simulink model "quadplane_controlA"  (R2023a)
settings: Solver=VariableStepAuto  StartTime=0.0  StopTime=10.0  RelTol=1e-3
undefined symbols (not defined in the file or in its folder): framePeriod_s
libraries: simulink x4
settings Model: Creator=lagerprocessor  LastModifiedBy=lagerprocessor

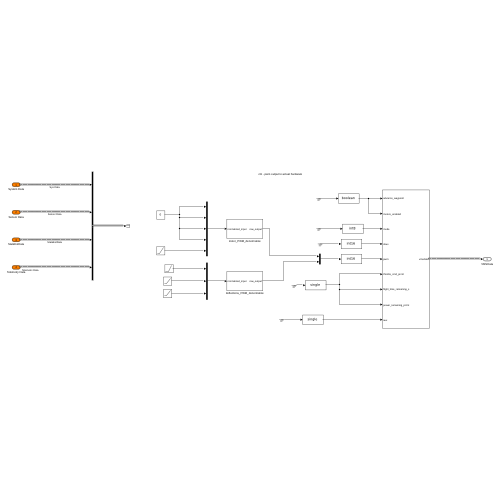
[thumbnail: Simulink's stored preview of the top-level diagram]
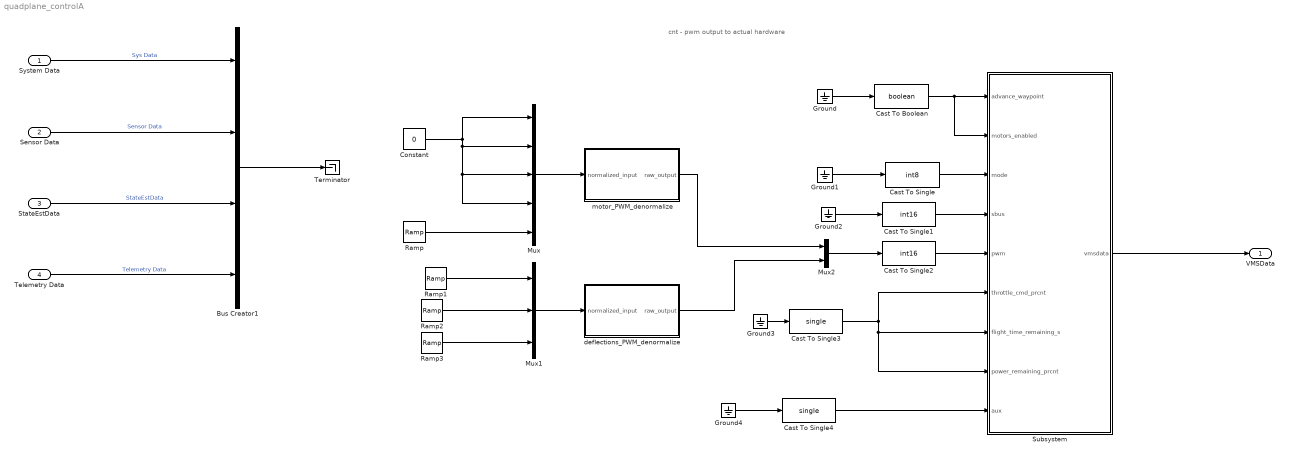
== system quadplane_controlA ==
  note: cnt - pwm output to actual hardware
  System Data : Inport  OutDataTypeStr=Bus: SysData  SampleTime=framePeriod_s  BusOutputAsStruct=on
  Sensor Data : Inport  Port=2  OutDataTypeStr=Bus: SensorData  SampleTime=framePeriod_s  BusOutputAsStruct=on
  StateEstData : Inport  Port=3  OutDataTypeStr=Bus: StateEstData  SampleTime=framePeriod_s  BusOutputAsStruct=on
  Telemetry Data : Inport  Port=4  OutDataTypeStr=Bus: TelemData  SampleTime=framePeriod_s  BusOutputAsStruct=on
  Bus Creator1 : BusCreator  Inputs=4
  Cast To Boolean : DataTypeConversion  OutDataTypeStr=boolean  SaturateOnIntegerOverflow=off  RndMeth=Floor
  Cast To Single : DataTypeConversion  OutDataTypeStr=int8  SaturateOnIntegerOverflow=off  RndMeth=Floor
  Cast To Single1 : DataTypeConversion  OutDataTypeStr=int16  SaturateOnIntegerOverflow=off  RndMeth=Floor
  Cast To Single2 : DataTypeConversion  OutDataTypeStr=int16  SaturateOnIntegerOverflow=off  RndMeth=Floor
  Cast To Single3 : DataTypeConversion  OutDataTypeStr=single  SaturateOnIntegerOverflow=off  RndMeth=Floor
  Cast To Single4 : DataTypeConversion  OutDataTypeStr=single  SaturateOnIntegerOverflow=off  RndMeth=Floor
  Constant : Constant  Value=0
  Ground{,1..4} (5 alike) : Ground
  Mux : Mux  Inputs=5
  Mux1 : Mux  Inputs=3
  Mux2 : Mux  Inputs=2
  Ramp : simulink/Sources/Ramp  slope=0  start=0  InitialOutput=0.4
  Ramp1 : simulink/Sources/Ramp  slope=0  start=0  InitialOutput=0
  Ramp2 : simulink/Sources/Ramp  slope=0  start=0  InitialOutput=0
  Ramp3 : simulink/Sources/Ramp  slope=0  start=0  InitialOutput=0
  Subsystem : Subsystem
  Terminator : Terminator
  deflections_PWM_denormalize : Subsystem
  motor_PWM_denormalize : Subsystem
  VMSData : Outport  OutDataTypeStr=Bus: VmsData
  wires:
  Telemetry Data/1 -> Bus Creator1/4  "Telemetry Data"
  StateEstData/1 -> Bus Creator1/3  "StateEstData"
  Sensor Data/1 -> Bus Creator1/2  "Sensor Data"
  System Data/1 -> Bus Creator1/1  "Sys Data"
  Bus Creator1/1 -> Terminator/1
  motor_PWM_denormalize/1(raw_output) -> Mux2/1
  Ground/1 -> Cast To Boolean/1
  Ground1/1 -> Cast To Single/1
  Ground2/1 -> Cast To Single1/1
  Cast To Single3/1 -> Subsystem/6(throttle_cmd_prcnt), Subsystem/8(power_remaining_prcnt), Subsystem/7(flight_time_remaining_s)
  Cast To Single4/1 -> Subsystem/9(aux)
  Subsystem/1(vmsdata) -> VMSData/1
  Cast To Boolean/1 -> Subsystem/2(motors_enabled), Subsystem/1(advance_waypoint)
  Cast To Single/1 -> Subsystem/3(mode)
  Cast To Single1/1 -> Subsystem/4(sbus)
  Cast To Single2/1 -> Subsystem/5(pwm)
  Ground3/1 -> Cast To Single3/1
  Ground4/1 -> Cast To Single4/1
  Mux/1 -> motor_PWM_denormalize/1(normalized_input)
  Ramp/1 -> Mux/5
  Constant/1 -> Mux/4, Mux/3, Mux/2, Mux/1
  Mux1/1 -> deflections_PWM_denormalize/1(normalized_input)
  deflections_PWM_denormalize/1(raw_output) -> Mux2/2
  Mux2/1 -> Cast To Single2/1
  Ramp3/1 -> Mux1/3
  Ramp2/1 -> Mux1/2
  Ramp1/1 -> Mux1/1

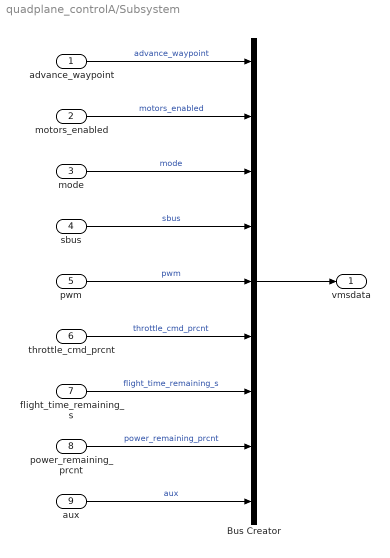
== system quadplane_controlA/Subsystem ==
  advance_waypoint : Inport
  motors_enabled : Inport  Port=2
  mode : Inport  Port=3
  sbus : Inport  Port=4
  pwm : Inport  Port=5
  throttle_cmd_prcnt : Inport  Port=6
  flight_time_remaining_s : Inport  Port=7
  power_remaining_prcnt : Inport  Port=8
  aux : Inport  Port=9
  Bus Creator : BusCreator  Inputs=9  OutDataTypeStr=Bus: VmsData  NonVirtualBus=on
      settings: InheritFromInputs=off
  vmsdata : Outport
  wires:
  flight_time_remaining_s/1 -> Bus Creator/7  "flight_time_remaining_s"
  mode/1 -> Bus Creator/3  "mode"
  pwm/1 -> Bus Creator/5  "pwm"
  aux/1 -> Bus Creator/9  "aux"
  throttle_cmd_prcnt/1 -> Bus Creator/6  "throttle_cmd_prcnt"
  Bus Creator/1 -> vmsdata/1
  motors_enabled/1 -> Bus Creator/2  "motors_enabled"
  advance_waypoint/1 -> Bus Creator/1  "advance_waypoint"
  power_remaining_prcnt/1 -> Bus Creator/8  "power_remaining_prcnt"
  sbus/1 -> Bus Creator/4  "sbus"

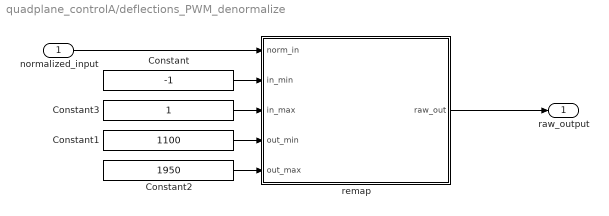
== system quadplane_controlA/deflections_PWM_denormalize ==
  normalized_input : Inport
  Constant : Constant  Value=-1  OutDataTypeStr=single
  Constant1 : Constant  Value=1100  OutDataTypeStr=single
  Constant2 : Constant  Value=1950  OutDataTypeStr=single
  Constant3 : Constant  OutDataTypeStr=single
  remap : MATLAB Function  TreatAsAtomicUnit=on
  raw_output : Outport
  wires:
  Constant2/1 -> remap/5(out_max)
  Constant1/1 -> remap/4(out_min)
  Constant3/1 -> remap/3(in_max)
  Constant/1 -> remap/2(in_min)
  remap/1(raw_out) -> raw_output/1
  normalized_input/1 -> remap/1(norm_in)

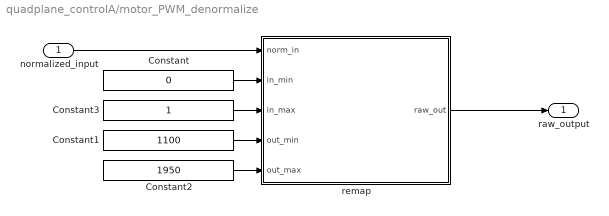
== system quadplane_controlA/motor_PWM_denormalize ==
  normalized_input : Inport
  Constant : Constant  Value=0  OutDataTypeStr=single
  Constant1 : Constant  Value=1100  OutDataTypeStr=single
  Constant2 : Constant  Value=1950  OutDataTypeStr=single
  Constant3 : Constant  OutDataTypeStr=single
  remap : MATLAB Function  TreatAsAtomicUnit=on
  raw_output : Outport
  wires:
  Constant2/1 -> remap/5(out_max)
  Constant1/1 -> remap/4(out_min)
  Constant3/1 -> remap/3(in_max)
  Constant/1 -> remap/2(in_min)
  remap/1(raw_out) -> raw_output/1
  normalized_input/1 -> remap/1(norm_in)

== matlab function quadplane_controlA/deflections_PWM_denormalize/remap ==
  data: norm_in input; raw_out output; in_min input; in_max input; out_min input; out_max input
function raw_out = remap(norm_in,in_min,in_max,out_min,out_max)
raw_out = (norm_in - in_min) * (out_max - out_min)/(in_max-in_min) + out_min;

== matlab function quadplane_controlA/motor_PWM_denormalize/remap ==
  data: norm_in input; raw_out output; in_min input; in_max input; out_min input; out_max input
function raw_out = remap(norm_in,in_min,in_max,out_min,out_max)
raw_out = (norm_in - in_min) * (out_max - out_min)/(in_max-in_min) + out_min;
